simulink model "Blokdiagram"  (R2019a)
settings: Solver=VariableStepAuto  StartTime=0.0  StopTime=3600  RelTol=1e-3
settings Model: Creator=Anton  LastModifiedBy=Anton

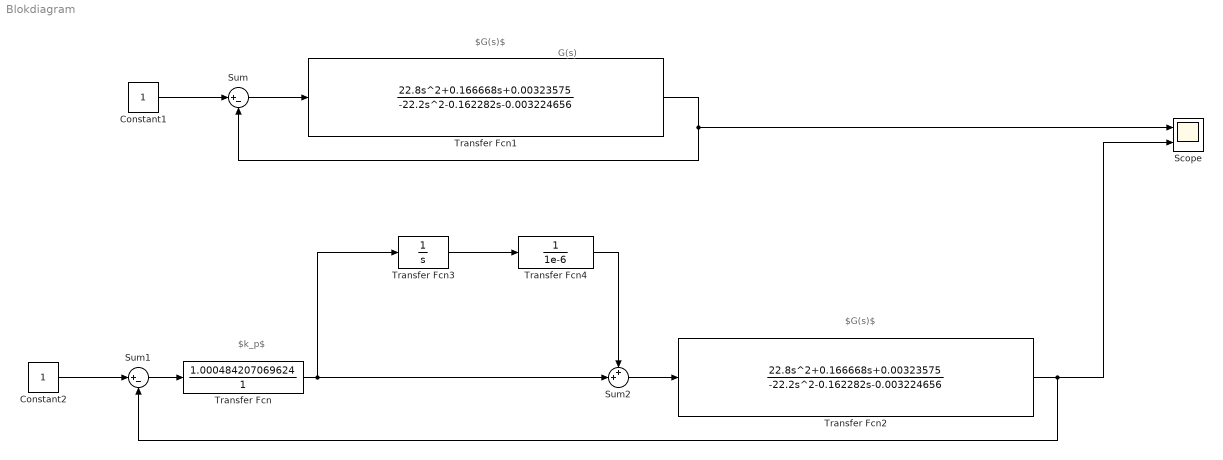
== system Blokdiagram ==
  note: $k_p$
  note: G(s)
  note: $G(s)$
  note: $G(s)$
  Constant1 : Constant
  Constant2 : Constant
  Scope : Scope  NumInputPorts=2
  Sum : Sum  Inputs=|+-
  Sum1 : Sum  Inputs=|+-
  Sum2 : Sum  Inputs=++|
  Transfer Fcn : TransferFcn  Numerator=[1.000484207069624]  Denominator=[1]
  Transfer Fcn1 : TransferFcn  Numerator=[22.8,0.166668,0.00323575]  Denominator=[-22.2,-0.162282,-0.003224656]
  Transfer Fcn2 : TransferFcn  Numerator=[22.8,0.166668,0.00323575]  Denominator=[-22.2,-0.162282,-0.003224656]
  Transfer Fcn3 : TransferFcn  Denominator=[1 0]
  Transfer Fcn4 : TransferFcn  Denominator=[1e-6]
  wires:
  Constant1/1 -> Sum/1
  Transfer Fcn1/1 -> Scope/1, Sum/2
  Sum/1 -> Transfer Fcn1/1
  Constant2/1 -> Sum1/1
  Sum1/1 -> Transfer Fcn/1
  Transfer Fcn/1 -> Sum2/2, Transfer Fcn3/1
  Transfer Fcn3/1 -> Transfer Fcn4/1
  Transfer Fcn4/1 -> Sum2/1
  Sum2/1 -> Transfer Fcn2/1
  Transfer Fcn2/1 -> Scope/2, Sum1/2
